simulink model "Adaptivecontroller"  (Simulink 7.5)
settings: Solver=ode15s  StartTime=0.0  StopTime=10.0  RelTol=1e-3
InitFcn:
  | traj_start
StopFcn:
  | displayarm
undefined symbols (not defined in the file or in its folder): Cmat_ad, Dmat_sim, Gmat_sim
settings Model: Creator=Prasad  LastModifiedBy=Prasad

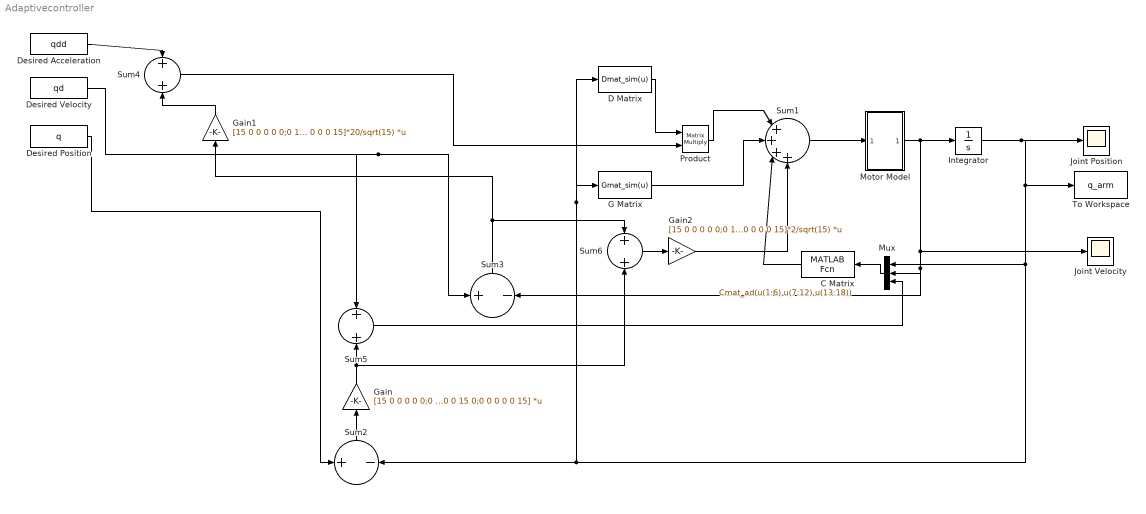
== system Adaptivecontroller ==
  C Matrix : MATLABFcn  MATLABFcn=Cmat_ad(u(1:6),u(7:12),u(13:18))  OutputSignalType=real  Output1D=off
  D Matrix : MATLABFcn  MATLABFcn=Dmat_sim(u)  OutputSignalType=real  Output1D=off
  Desired Acceleration : FromWorkspace  VariableName=qdd  SampleTime=0  OutputAfterFinalValue=Holding final value
  Desired Position : FromWorkspace  VariableName=q  SampleTime=0  OutputAfterFinalValue=Holding final value
  Desired Velocity : FromWorkspace  VariableName=qd  SampleTime=0  OutputAfterFinalValue=Holding final value
  G Matrix : MATLABFcn  MATLABFcn=Gmat_sim(u)  OutputSignalType=real  Output1D=off
  Gain : Gain  Gain=[15 0 0 0 0 0;0 15 0 0 0 0;0 0 15 0 0 0;0 0 0 15 0 0;0 0 0 0 15 0;0 0 0 0 0 15]  Multiplication=Matrix(K*u)  ParameterDataType=fixdt(1, 16)  ParameterScaling=2^0  OutDataType=fixdt(1, 16)  OutScaling=2^0
  Gain1 : Gain  Gain=[15 0 0 0 0 0;0 15 0 0 0 0;0 0 15 0 0 0;0 0 0 15 0 0;0 0 0 0 15 0;0 0 0 0 0 15]*20/sqrt(15)  Multiplication=Matrix(K*u)  ParameterDataType=fixdt(1, 16)  ParameterScaling=2^0  OutDataType=fixdt(1, 16)  OutScaling=2^0
  Gain2 : Gain  Gain=[15 0 0 0 0 0;0 15 0 0 0 0;0 0 15 0 0 0;0 0 0 15 0 0;0 0 0 0 15 0;0 0 0 0 0 15]*2/sqrt(15)  Multiplication=Matrix(K*u)  ParameterDataType=fixdt(1, 16)  ParameterScaling=2^0  OutDataType=fixdt(1, 16)  OutScaling=2^0
  Integrator : Integrator  InitialCondition=[1 1 1 1 1 1]
  Joint Position : Scope
      settings: TimeRange=10  YMin=0.1  YMax=0.6
  Joint Velocity : Scope
      settings: TimeRange=10  YMin=-18  YMax=2
  Motor Model : Subsystem
  Mux : Mux  Inputs=3
  Product : Product  Multiplication=Matrix(*)  OutDataType=fixdt(1, 16)  OutScaling=2^0  RndMeth=Zero
  Sum1 : Sum  Inputs=|++++  OutDataType=fixdt(1, 16)  OutScaling=2^0
  Sum2 : Sum  Inputs=+|-  OutDataType=fixdt(1, 16)  OutScaling=2^0
  Sum3 : Sum  Inputs=+-  OutDataType=fixdt(1, 16)  OutScaling=2^0
  Sum4 : Sum  Inputs=+|+  OutDataType=fixdt(1, 16)  OutScaling=2^0
  Sum5 : Sum  Inputs=+|+  OutDataType=fixdt(1, 16)  OutScaling=2^0
  Sum6 : Sum  Inputs=+|+  OutDataType=fixdt(1, 16)  OutScaling=2^0
  To Workspace : ToWorkspace  VariableName=q_arm  SampleTime=-1  SaveFormat=Structure
  wires:
  D Matrix/1 -> Product/1
  G Matrix/1 -> Sum1/2
  Product/1 -> Sum1/1
  C Matrix/1 -> Sum1/3
  Sum1/1 -> Motor Model/1(In1)
  Motor Model/1(Out1) -> Joint Velocity/1, Mux/2, Sum3/2, Integrator/1
  Integrator/1 -> Joint Position/1, Sum2/2, D Matrix/1, G Matrix/1, Mux/1, To Workspace/1
  Mux/1 -> C Matrix/1
  Desired Velocity/1 -> Sum3/1, Sum5/1
  Desired Position/1 -> Sum2/1
  Desired Acceleration/1 -> Sum4/1
  Gain1/1 -> Sum4/2
  Sum2/1 -> Gain/1
  Gain/1 -> Sum5/2, Sum6/2
  Sum5/1 -> Mux/3
  Sum4/1 -> Product/2
  Sum3/1 -> Gain1/1, Sum6/1
  Sum6/1 -> Gain2/1
  Gain2/1 -> Sum1/4

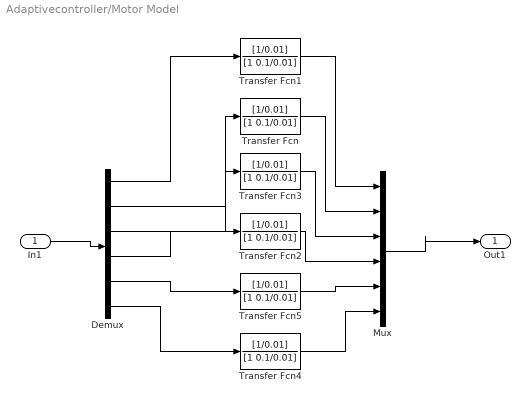
== system Adaptivecontroller/Motor Model ==
  In1 : Inport
  Demux : Demux  Outputs=6
  Mux : Mux  Inputs=6
  Transfer Fcn{,1..5} (6 alike) : TransferFcn  Numerator=[1/0.01]  Denominator=[1 0.1/0.01]
  Out1 : Outport
  wires:
  Mux/1 -> Out1/1
  Transfer Fcn4/1 -> Mux/6
  Transfer Fcn5/1 -> Mux/5
  Transfer Fcn2/1 -> Mux/4
  Transfer Fcn3/1 -> Mux/3
  Transfer Fcn/1 -> Mux/2
  Transfer Fcn1/1 -> Mux/1
  Demux/6 -> Transfer Fcn4/1
  Demux/5 -> Transfer Fcn5/1
  Demux/4 -> Transfer Fcn2/1
  Demux/3 -> Transfer Fcn3/1
  Demux/2 -> Transfer Fcn/1
  Demux/1 -> Transfer Fcn1/1
  In1/1 -> Demux/1
